simulink model "test"  (R2022b)
settings: Solver=VariableStepAuto  StartTime=0.0  StopTime=10.0  RelTol=1e-3
libraries: simulink x2, hdlsllib x2
settings Model: Creator=padlewsk  LastModifiedBy=padlewsk

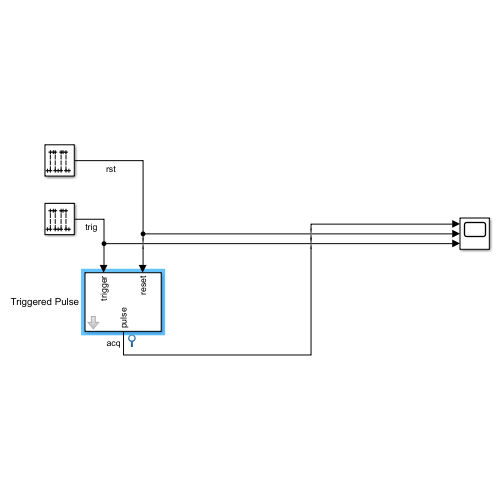
[thumbnail: Simulink's stored preview of the top-level diagram]
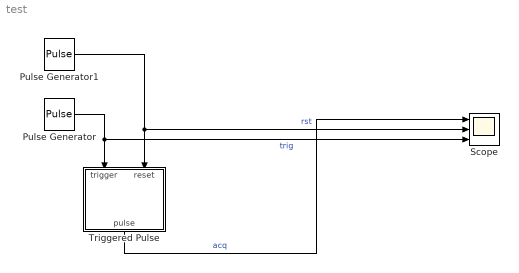
== system test ==
  Pulse Generator : DiscretePulseGenerator  Period=1e100  PhaseDelay=5  SampleTime=0.1
  Pulse Generator1 : DiscretePulseGenerator  Period=1e100  PhaseDelay=10  SampleTime=0.1
  Scope : Scope  NumInputPorts=3
  Triggered Pulse : Subsystem  mask(Triggered Pulse){N=3}
      mask prompts: N "Length (N samples)"
      mask help: Generates a single pulse of N samples length
  wires:
  Triggered Pulse/1(pulse) -> Scope/1  "acq"
  Pulse Generator/1 -> Triggered Pulse/1(trigger), Scope/3  "trig"
  Pulse Generator1/1 -> Scope/2, Triggered Pulse/2(reset)  "rst"

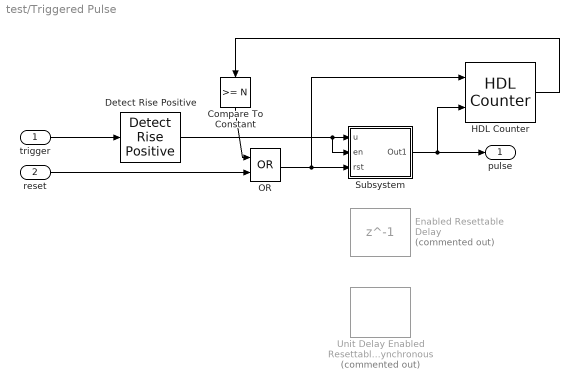
== system test/Triggered Pulse ==
  trigger : Inport
  reset : Inport  Port=2
  Compare To Constant : simulink/Logic and Bit Operations/Compare To Constant  relop=>=  const=N  OutDataTypeStr=boolean
  Detect Rise Positive : simulink/Logic and Bit Operations/Detect Rise Positive  vinit=0  OutDataTypeStr=boolean
  Enabled Resettable Delay : Delay  Commented=on  DelayLength=1  ExternalReset=Level hold  ShowEnablePort=on
      settings: InputPortMap=u0,e6,r5
  HDL Counter : hdlsllib/Sources/HDL Counter  CountType=Free running  CountInit=1  CountStep=1  CountMax=25  CountFromType=Initial value  CountFrom=1  CountResetPort=on  CountLoadPort=off  CountEnbPort=on  CountDirPort=off  CountHitOutputPort=off  CountDataType=Unsigned  CountWordLen=32  CountFracLen=0  CountSampTime=1
  OR : Logic  Operator=OR  AllPortsSameDT=off  OutDataTypeStr=boolean
  Subsystem : Subsystem
  Unit Delay Enabled Resettable Synchronous : hdlsllib/Discrete/Unit Delay Enabled Resettable Synchronous  Commented=on  InitialCondition=0.0  SampleTime=-1
  pulse : Outport  VectorParamsAs1DForOutWhenUnconnected=off
  wires:
  OR/1 -> Subsystem/3(rst), HDL Counter/1
  trigger/1 -> Detect Rise Positive/1
  Subsystem/1(Out1) -> HDL Counter/2, pulse/1
  Compare To Constant/1 -> OR/1
  reset/1 -> OR/2
  Detect Rise Positive/1 -> Subsystem/2(en), Subsystem/1(u)
  HDL Counter/1 -> Compare To Constant/1

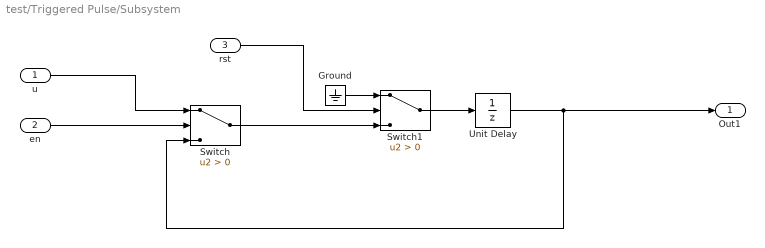
== system test/Triggered Pulse/Subsystem ==
  u : Inport
  en : Inport  Port=2
  rst : Inport  Port=3
  Ground : Ground
  Switch : Switch  Criteria=u2 > Threshold  SaturateOnIntegerOverflow=off  InputSameDT=off
  Switch1 : Switch  Criteria=u2 > Threshold  SaturateOnIntegerOverflow=off  InputSameDT=off
  Unit Delay : UnitDelay  SampleTime=-1  HasFrameUpgradeWarning=on
  Out1 : Outport
  wires:
  Unit Delay/1 -> Switch/3, Out1/1
  en/1 -> Switch/2
  u/1 -> Switch/1
  rst/1 -> Switch1/2
  Ground/1 -> Switch1/1
  Switch1/1 -> Unit Delay/1
  Switch/1 -> Switch1/3
